simulink model "Utilization_Model"  (R2023a)
settings: Solver=VariableStepAuto  StartTime=0.0  StopTime=10.0  RelTol=1e-3
libraries: NSA_DEVS_SINKS_ATOMIC x5, NSA_DEVS_LOGISTICS_ATOMIC x3, NSA_DEVS_SOURCES_ATOMIC x1, NSA_DEVS_STATISTICS_ATOMIC x1
settings Model: Creator=david  LastModifiedBy=david

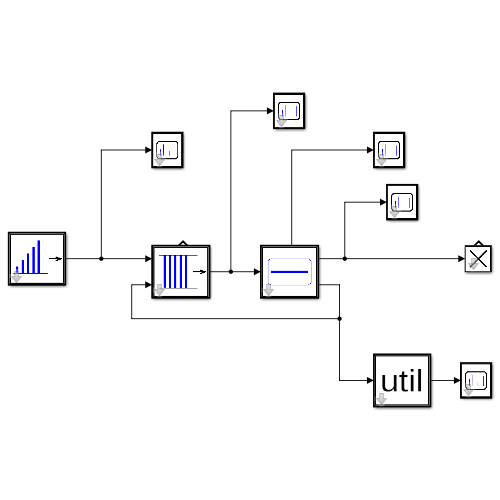
[thumbnail: Simulink's stored preview of the top-level diagram]
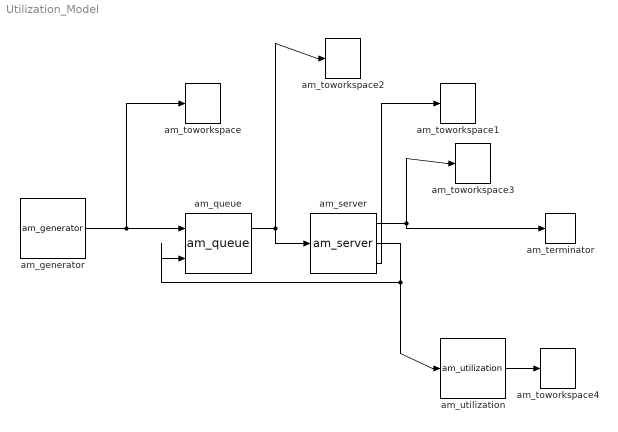
== system Utilization_Model ==
  am_generator : NSA_DEVS_SOURCES_ATOMIC/am_generator  tG=6  n0=1  nG=1000  tau=[0,1]  debug=0
      settings: SourceProductName=NSA_DEVS
  am_queue : NSA_DEVS_LOGISTICS_ATOMIC/am_queue  tD=[0,2]  tau=[0,2]  debug=0
      settings: SourceProductName=NSA_DEVS
  am_server : NSA_DEVS_LOGISTICS_ATOMIC/am_server  tS=1.5  tau=[0,1]  debug=0
      settings: SourceProductName=NSA_DEVS
  am_terminator : NSA_DEVS_LOGISTICS_ATOMIC/am_terminator  tau=[0,1]  debug=0
      settings: SourceProductName=NSA_DEVS
  am_toworkspace : NSA_DEVS_SINKS_ATOMIC/am_toworkspace  varname="\"genOut\""  t0=0  format="\"vector\""  tau=[0,5]  debug=0
      settings: SourceProductName=NSA_DEVS
  am_toworkspace1 : NSA_DEVS_SINKS_ATOMIC/am_toworkspace  varname="\"srvnOut\""  t0=0  format="\"vector\""  tau=[0,5]  debug=0
      settings: SourceProductName=NSA_DEVS
  am_toworkspace2 : NSA_DEVS_SINKS_ATOMIC/am_toworkspace  varname="\"queOut\""  t0=0  format="\"vector\""  tau=[0,5]  debug=0
      settings: SourceProductName=NSA_DEVS
  am_toworkspace3 : NSA_DEVS_SINKS_ATOMIC/am_toworkspace  varname="\"srvOut\""  t0=0  format="\"vector\""  tau=[0,5]  debug=0
      settings: SourceProductName=NSA_DEVS
  am_toworkspace4 : NSA_DEVS_SINKS_ATOMIC/am_toworkspace  varname="\"utilOut\""  t0=0  format="\"vector\""  tau=[0,5]  debug=0
      settings: SourceProductName=NSA_DEVS
  am_utilization : NSA_DEVS_STATISTICS_ATOMIC/am_utilization  tau=[0,1]  debug=0
      settings: SourceProductName=NSA_DEVS
  wires:
  am_generator/1 -> am_toworkspace/1, am_queue/1
  am_queue/1 -> am_toworkspace2/1, am_server/1
  am_server/2 -> am_utilization/1, am_queue/2
  am_server/1 -> am_toworkspace3/1, am_terminator/1
  am_utilization/1 -> am_toworkspace4/1
  am_server/3 -> am_toworkspace1/1
